simulink model "te_14_4_22_es2_sim"  (R2023a)
settings: Solver=VariableStepAuto  StartTime=0.0  StopTime=10.0  RelTol=1e-3
values from neighbouring files (symbols this model uses):
  Clin = [1 0]    [te_14_1_22_es2.m]
  K = place(Alin,Blin,[a1,2*a1])    [te_14_1_22_es2.m]
  x0 = [3;5]    [te_14_1_22_es2.m]
settings Model: Creator=Admin  LastModifiedBy=Admin

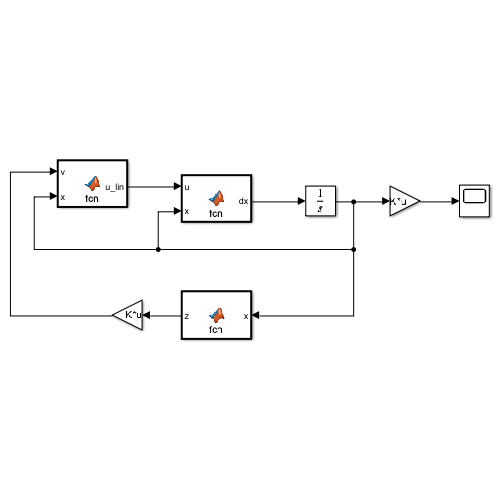
[thumbnail: Simulink's stored preview of the top-level diagram]
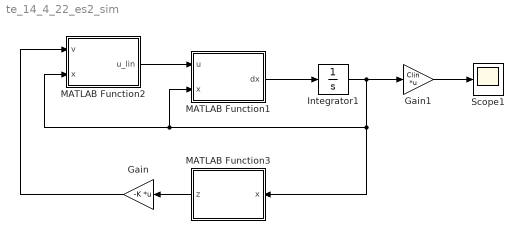
== system te_14_4_22_es2_sim ==
  Gain : Gain  Gain=-K  Multiplication=Matrix(K*u)
  Gain1 : Gain  Gain=Clin  Multiplication=Matrix(K*u)
  Integrator1 : Integrator  InitialCondition=x0
  MATLAB Function1 : MATLAB Function  TreatAsAtomicUnit=on
  MATLAB Function2 : MATLAB Function  TreatAsAtomicUnit=on
  MATLAB Function3 : MATLAB Function  TreatAsAtomicUnit=on
  Scope1 : Scope
  wires:
  MATLAB Function1/1(dx) -> Integrator1/1
  Integrator1/1 -> Gain1/1, MATLAB Function2/2(x), MATLAB Function1/2(x), MATLAB Function3/1(x)
  MATLAB Function2/1(u_lin) -> MATLAB Function1/1(u)
  MATLAB Function3/1(z) -> Gain/1
  Gain/1 -> MATLAB Function2/1(v)
  Gain1/1 -> Scope1/1

== matlab function te_14_4_22_es2_sim/MATLAB Function2 ==
  data: v input; u_lin output; x input
function u_lin = fcn(v,x)
x1=x(1);
x2=x(2);
u_lin=((3*x1 - 3*x2)*(x1^2 + x1) - v + (x2^2*(6*x1 + 3)*(3*x1^2 + 3*x1))/3)/((3*x2 - 18)*(x1^2 + x1));

== matlab function te_14_4_22_es2_sim/MATLAB Function3 ==
  data: z output; x input
function z = fcn(x)
x1=x(1);
x2=x(2);

z=[x1/3; (x2*(3*x1^2 + 3*x1))/3];

== matlab function te_14_4_22_es2_sim/MATLAB Function1 ==
  data: u input; dx output; x input
function dx = fcn(u,x)
x1=x(1);
x2=x(2);
dx=[3*(x1^2+x1)*x2;-3*x2+3*x1-3*x2*u+18*u];
